simulink model "demo"  (R2021b)
settings: Solver=VariableStepAuto  StartTime=0.0  StopTime=10.0  RelTol=1e-3
values from neighbouring files (symbols this model uses):
  sortedParams = table2struct(sortedT)    [Experiment.m]
settings Model: Creator=liuqingyang  LastModifiedBy=liuqingyang

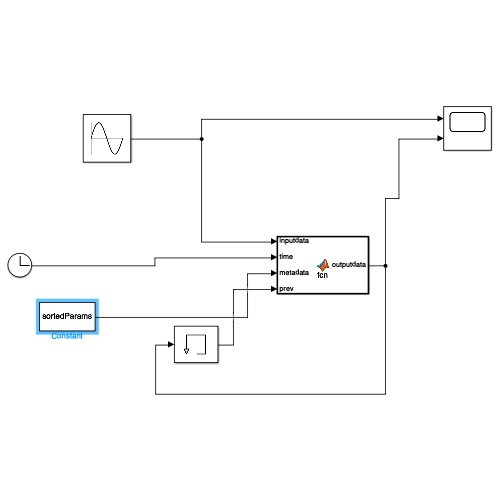
[thumbnail: Simulink's stored preview of the top-level diagram]
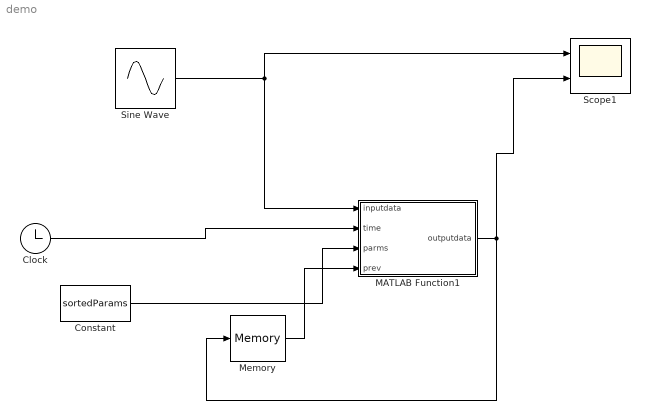
== system demo ==
  Clock : Clock
  Constant : Constant  Value=sortedParams  OutDataTypeStr=Bus:slBus1
  MATLAB Function1 : MATLAB Function  TreatAsAtomicUnit=on
  Memory : Memory
  Scope1 : Scope  NumInputPorts=2
  Sine Wave : Sin  Amplitude=10  Frequency=2  Samples=1000000  SampleTime=0
  wires:
  MATLAB Function1/1(outputdata) -> Memory/1, Scope1/2
  Sine Wave/1 -> MATLAB Function1/1(inputdata), Scope1/1
  Clock/1 -> MATLAB Function1/2(time)
  Memory/1 -> MATLAB Function1/4(prev)
  Constant/1 -> MATLAB Function1/3(parms)

== matlab function demo/MATLAB Function1 ==
  data: inputdata input; outputdata output; time input; parms input; prev input

function outputdata = fcn(inputdata, time, parms, prev)

% default
outputdata = inputdata;

for i = 1 : length(parms)

    if time < parms(i).StartTime 
        break;
    elseif time > parms(i).EndTime 
        continue;
    else
       switch parms(i).InjectionType
        case 1
           inject1 = SuddenInjection(parms(i).Val);
           outputdata = injection(inject1, inputdata);
        case 2 
           inject2 = DeltaInjection(parms(i).Val);
           outputdata = injection(inject2, inputdata);
           otherwise
           inject3 = GradualInjection(parms(i).Type, parms(i).Coef1, parms(i).Coef2, parms(i).Freq, time);
           outputdata = injection(inject3, prev);
        end
    end

end

end
